simulink model "TRNG_test03"  (R2020a)
settings: Solver=VariableStepAuto  StartTime=0.0  StopTime=10.0  RelTol=1e-3
undefined symbols (not defined in the file): AXI4, Lite
libraries: xbsIndex_r4 x48
settings Model: Creator=ringl  LastModifiedBy=ringl

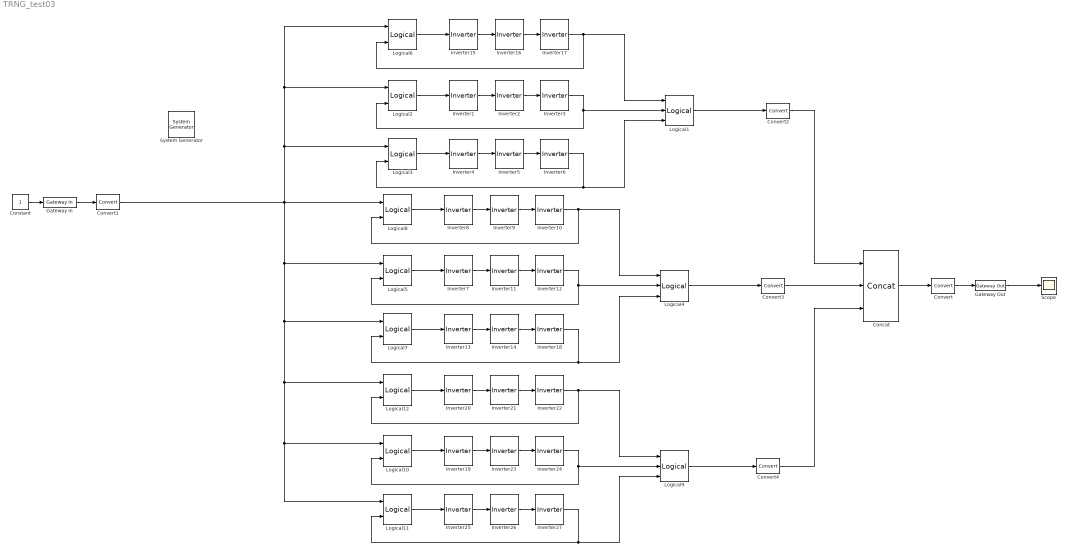
== system TRNG_test03 ==
  " System Generator" : xbsIndex_r4/ System Generator  Tag=genX  xilinxfamily=zynq  part=xc7z020  speed=-1  package=clg400  synthesis_tool=Vivado  clock_wrapper=Clock Enables  directory=./netlist  proj_type=Vivado  Synth_file=Vivado Synthesis Defaults  Impl_file=Vivado Implementation Defaults  testbench=off  simulink_period=1  sysclk_period=10  dcm_input_clock_period=10  incr_netlist=off  trim_vbits=Everywhere in SubSystem  dbl_ovrd=According to Block Masks  core_generation=According to Block Masks  run_coregen=off  deprecated_control=off  eval_field=0  block_type=sysgen
  Concat : xbsIndex_r4/Concat  num_inputs=3  dbl_ovrd=off  block_type=concat
  Constant : Constant
  Convert : xbsIndex_r4/Convert  gui_display_data_type=Fixed-point  arith_type="Signed  (2's comp)"  n_bits=32  bin_pt=0  float_type=Single  exp_bits=8  fraction_bits=24  quantization=Truncate  overflow=Wrap  en=off  latency=1  pipeline=off  dbl_ovrd=off  block_type=convert
  Convert1 : xbsIndex_r4/Convert  gui_display_data_type=Fixed-point  arith_type="Signed  (2's comp)"  n_bits=1  bin_pt=0  float_type=Single  exp_bits=8  fraction_bits=24  quantization=Truncate  overflow=Wrap  en=off  latency=1  pipeline=off  dbl_ovrd=off  block_type=convert
  Convert2 : xbsIndex_r4/Convert  gui_display_data_type=Fixed-point  arith_type=Unsigned  n_bits=1  bin_pt=0  float_type=Single  exp_bits=8  fraction_bits=24  quantization=Truncate  overflow=Wrap  en=off  latency=1  pipeline=off  dbl_ovrd=off  block_type=convert
  Convert3 : xbsIndex_r4/Convert  gui_display_data_type=Fixed-point  arith_type=Unsigned  n_bits=1  bin_pt=0  float_type=Single  exp_bits=8  fraction_bits=24  quantization=Truncate  overflow=Wrap  en=off  latency=1  pipeline=off  dbl_ovrd=off  block_type=convert
  Convert4 : xbsIndex_r4/Convert  gui_display_data_type=Fixed-point  arith_type=Unsigned  n_bits=1  bin_pt=0  float_type=Single  exp_bits=8  fraction_bits=24  quantization=Truncate  overflow=Wrap  en=off  latency=1  pipeline=off  dbl_ovrd=off  block_type=convert
  Gateway In : xbsIndex_r4/Gateway In  gui_display_data_type=Fixed-point  arith_type="Signed  (2's comp)"  n_bits=32  bin_pt=0  preci_type=Single  exp_width=8  frac_width=24  rows=1  columns=1  quantization="Round  (unbiased: +/- Inf)"  overflow=Saturate  period=1  UseAsADC=off  ADCChannel='1'  interface=AXI4-Lite  automatic_assignment=on  address_offset=hex2dec('00')  intf_name=''  intf_description=''  default_value=0  timing_constraint=None  locs_specified=off  LOCs={}  io_standard={}  inherit_from_input=off  hdl_port=on  dbl_ovrd=off  block_type=gatewayin
  Gateway Out : xbsIndex_r4/Gateway Out  inherit_from_input=off  hdl_port=on  rows=1  columns=1  UseAsDAC=off  DACChannel='1'  interface=AXI4-Lite  automatic_assignment=on  address_offset=hex2dec('00')  intf_name=''  intf_description=''  timing_constraint=None  locs_specified=off  LOCs={}  io_standard={}  block_type=gatewayout
  Inverter{1..27} (27 alike) : xbsIndex_r4/Inverter  en=off  latency=1  dbl_ovrd=off  block_type=inv
  Logical1 : xbsIndex_r4/Logical  logical_function=XOR  inputs=3  en=off  latency=1  precision=Full  arith_type=Unsigned  n_bits=16  bin_pt=0  align_bp=on  dbl_ovrd=off  block_type=logical
  Logical{2..3,5..8,10..12} (9 alike) : xbsIndex_r4/Logical  logical_function=AND  inputs=2  en=off  latency=1  precision=Full  arith_type=Unsigned  n_bits=16  bin_pt=0  align_bp=on  dbl_ovrd=off  block_type=logical
  Logical4 : xbsIndex_r4/Logical  logical_function=XOR  inputs=3  en=off  latency=1  precision=Full  arith_type=Unsigned  n_bits=16  bin_pt=0  align_bp=on  dbl_ovrd=off  block_type=logical
  Logical9 : xbsIndex_r4/Logical  logical_function=XOR  inputs=3  en=off  latency=1  precision=Full  arith_type=Unsigned  n_bits=16  bin_pt=0  align_bp=on  dbl_ovrd=off  block_type=logical
  Scope : Scope
  wires:
  Inverter15/1 -> Inverter16/1
  Logical6/1 -> Inverter15/1
  Inverter17/1 -> Logical1/1, Logical6/2
  Inverter16/1 -> Inverter17/1
  Gateway In/1 -> Convert1/1
  Constant/1 -> Gateway In/1
  Concat/1 -> Convert/1
  Convert/1 -> Gateway Out/1
  Gateway Out/1 -> Scope/1
  Inverter2/1 -> Inverter3/1
  Inverter1/1 -> Inverter2/1
  Logical2/1 -> Inverter1/1
  Inverter3/1 -> Logical2/2, Logical1/2
  Inverter5/1 -> Inverter6/1
  Inverter4/1 -> Inverter5/1
  Logical3/1 -> Inverter4/1
  Inverter6/1 -> Logical1/3, Logical3/2
  Inverter8/1 -> Inverter9/1
  Inverter12/1 -> Logical5/2, Logical4/2
  Inverter7/1 -> Inverter11/1
  Inverter9/1 -> Inverter10/1
  Logical5/1 -> Inverter7/1
  Inverter11/1 -> Inverter12/1
  Inverter13/1 -> Inverter14/1
  Inverter14/1 -> Inverter18/1
  Logical8/1 -> Inverter8/1
  Inverter10/1 -> Logical4/1, Logical8/2
  Inverter18/1 -> Logical4/3, Logical7/2
  Logical7/1 -> Inverter13/1
  Inverter20/1 -> Inverter21/1
  Inverter24/1 -> Logical10/2, Logical9/2
  Inverter19/1 -> Inverter23/1
  Inverter21/1 -> Inverter22/1
  Logical10/1 -> Inverter19/1
  Inverter23/1 -> Inverter24/1
  Inverter25/1 -> Inverter26/1
  Inverter26/1 -> Inverter27/1
  Logical12/1 -> Inverter20/1
  Inverter22/1 -> Logical9/1, Logical12/2
  Inverter27/1 -> Logical9/3, Logical11/2
  Logical11/1 -> Inverter25/1
  Convert1/1 -> Logical11/1, Logical10/1, Logical12/1, Logical7/1, Logical5/1, Logical3/1, Logical2/1, Logical6/1, Logical8/1
  Convert2/1 -> Concat/1
  Convert3/1 -> Concat/2
  Convert4/1 -> Concat/3
  Logical4/1 -> Convert3/1
  Logical9/1 -> Convert4/1
  Logical1/1 -> Convert2/1
